simulink model "q2"  (R2020b)
settings: Solver=VariableStepAuto  StartTime=0.0  StopTime=100.0  RelTol=1e-3
PreLoadFcn:
  | start_time=0
  | sampling_time=0.1
  | end_time=100
  | m1=1200
  | k1=21000
  | b=2500
  | m2=13
  | k2=320
settings Model: Creator=Ravi  LastModifiedBy=Ravi

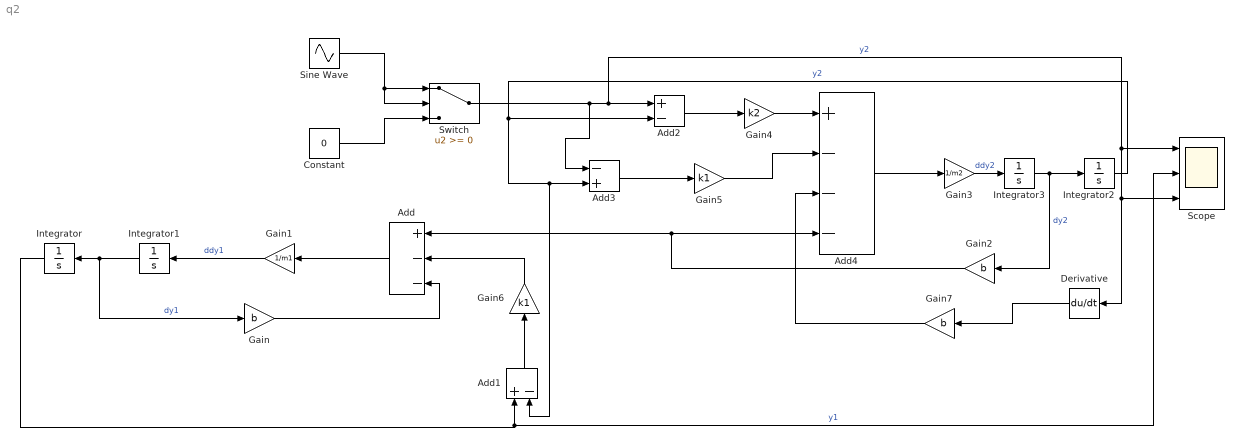
== system q2 ==
  Add : Sum  Inputs=+--
  Add1 : Sum  Inputs=+-
  Add2 : Sum  Inputs=+-
  Add3 : Sum  Inputs=-+
  Add4 : Sum  Inputs=+---
  Constant : Constant  Value=0
  Derivative : Derivative
  Gain : Gain  Gain=b
  Gain1 : Gain  Gain=1/m1
  Gain2 : Gain  Gain=b
  Gain3 : Gain  Gain=1/m2
  Gain4 : Gain  Gain=k2
  Gain5 : Gain  Gain=k1
  Gain6 : Gain  Gain=k1
  Gain7 : Gain  Gain=b
  Integrator{,1..3} (4 alike) : Integrator
  Scope : Scope  NumInputPorts=3
  Sine Wave : Sin  Frequency=0.1  SampleTime=0
  Switch : Switch
  wires:
  Gain1/1 -> Integrator1/1  "ddy1"
  Integrator1/1 -> Gain/1, Integrator/1  "dy1"
  Add/1 -> Gain1/1
  Gain6/1 -> Add/2
  Add1/1 -> Gain6/1
  Integrator/1 -> Scope/2, Add1/1  "y1"
  Constant/1 -> Switch/3
  Sine Wave/1 -> Switch/1, Switch/2
  Gain/1 -> Add/3
  Add4/1 -> Gain3/1
  Gain3/1 -> Integrator3/1  "ddy2"
  Integrator3/1 -> Gain2/1, Integrator2/1  "dy2"
  Gain2/1 -> Add/1, Add4/4
  Gain7/1 -> Add4/3
  Derivative/1 -> Gain7/1
  Add2/1 -> Gain4/1
  Gain4/1 -> Add4/1
  Gain5/1 -> Add4/2
  Add3/1 -> Gain5/1
  Integrator2/1 -> Add2/2, Add3/2, Add1/2  "y2"
  Switch/1 -> Add3/1, Scope/1, Scope/3, Derivative/1, Add2/1  "y2"
